simulink library "Aero_Model_Lib"  (R2019b)
settings: Solver=VariableStepAuto  StartTime=0.0  StopTime=10.0  RelTol=1e-3
settings Model: Creator=creal  LastModifiedBy=creal

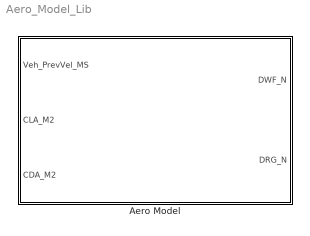
== system Aero_Model_Lib ==
  Aero Model : Subsystem

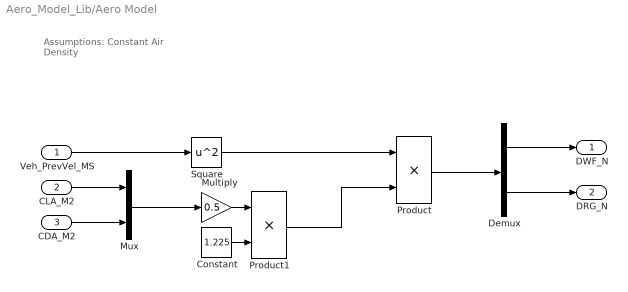
== system Aero_Model_Lib/Aero Model ==
  note: Assumptions:
      | Constant Air Density
  Veh_PrevVel_MS : Inport
  CLA_M2 : Inport  Port=2
  CDA_M2 : Inport  Port=3
  Constant : Constant  Value=1.225
  Demux : Demux  Outputs=2
  Multiply : Gain  Gain=0.5
  Mux : Mux  Inputs=2
  Product : Product
  Product1 : Product
  Square : Math  Operator=square  RndMeth=Zero  SaturateOnIntegerOverflow=on
  DWF_N : Outport
  DRG_N : Outport  Port=2
  wires:
  Mux/1 -> Multiply/1
  CLA_M2/1 -> Mux/1
  CDA_M2/1 -> Mux/2
  Veh_PrevVel_MS/1 -> Square/1
  Square/1 -> Product/1
  Multiply/1 -> Product1/1
  Constant/1 -> Product1/2
  Product1/1 -> Product/2
  Product/1 -> Demux/1
  Demux/1 -> DWF_N/1
  Demux/2 -> DRG_N/1
